simulink model "Compensador_Linealizacion_aproximada_del_RAP"  (R2022a)
settings: Solver=VariableStepAuto  StartTime=0.0  StopTime=10.0  RelTol=1e-3
libraries: cstblocks x2
settings Model: Creator=danie  LastModifiedBy=danie

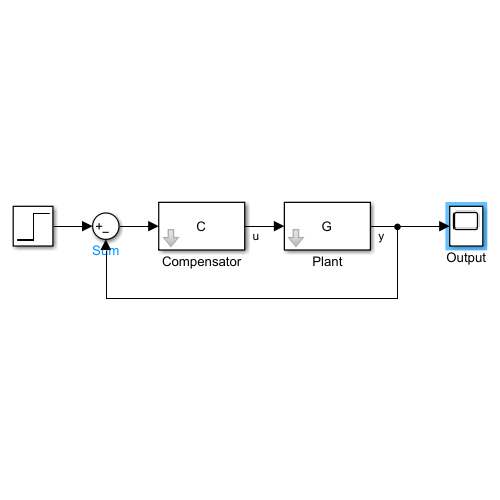
[thumbnail: Simulink's stored preview of the top-level diagram]
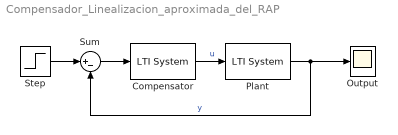
== system Compensador_Linealizacion_aproximada_del_RAP ==
  Compensator : cstblocks/LTI System  sys=C  IC=[]
  Output : Scope
  Plant : cstblocks/LTI System  sys=G  IC=[]
  Step : Step  SampleTime=0
  Sum : Sum  Inputs=|+-
  wires:
  Sum/1 -> Compensator/1
  Compensator/1 -> Plant/1  "u"
  Plant/1 -> Sum/2, Output/1  "y"
  Step/1 -> Sum/1
